simulink model "model_main2"  (R2024b)
settings: Solver=ode4  StartTime=0.0  StopTime=30  FixedStep=0.01  RelTol=1e-3
undefined symbols (not defined in the file): Iws, m_tot, Omega1_init, Omega2_init, Omega3_init, Omega4_init, pI0, qb0, RW_As, SC_Ib, SC_Kepler, TC_Kepler, vI0, wb0
libraries: simulink_extras x3, sharedtransform x2
settings Model: PacingRate=1.100000  Creator=yhj2019  LastModifiedBy=ASCL
settings RTWCC: GPUComputeCapability=3.5

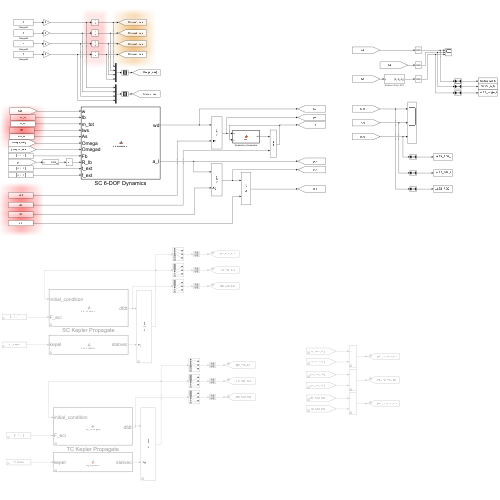
[thumbnail: Simulink's stored preview of the top-level diagram]
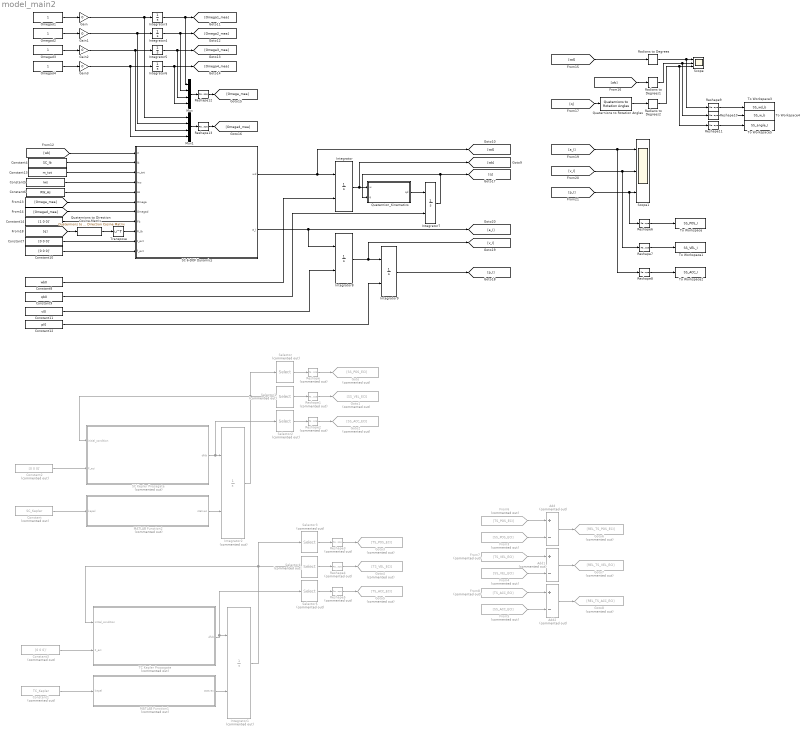
== system model_main2 ==
  Add : Sum  Commented=on  Inputs=+-
  Add1 : Sum  Commented=on  Inputs=+-
  Add2 : Sum  Commented=on  Inputs=+-
  Constant : Constant  Commented=on  Value=SC_Kepler
  Constant1 : Constant  Commented=on  Value=TC_Kepler
  Constant10 : Constant  Value=[0 0 0]'
  Constant11 : Constant  Value=vI0
  Constant12 : Constant  Value=pI0
  Constant13 : Constant  Value=m_tot
  Constant14 : Constant  Value=[1 0 0]'
  Constant2 : Constant  Commented=on  Value=[0 0 0]'
  Constant3 : Constant  Commented=on  Value=[0 0 0]'
  Constant4 : Constant  Value=SC_Ib
  Constant5 : Constant  Value=Iws
  Constant6 : Constant  Value=RW_As
  Constant7 : Constant  Value=[0 0 0]'
  Constant8 : Constant  Value=wb0
  Constant9 : Constant  Value=qb0
  From3 : From  Commented=on  GotoTag=SS_POS_ECI
  From4 : From  Commented=on  GotoTag=SS_VEL_ECI
  From5 : From  Commented=on  GotoTag=SS_ACC_ECI
  From6 : From  Commented=on  GotoTag=TS_POS_ECI
  From7 : From  Commented=on  GotoTag=TS_VEL_ECI
  From8 : From  Commented=on  GotoTag=TS_ACC_ECI
  Gain{,1..3} (4 alike) : Gain  Gain=0
  Goto : Goto  Commented=on  GotoTag=SS_POS_ECI
  Goto1 : Goto  Commented=on  GotoTag=SS_VEL_ECI
  Goto2 : Goto  Commented=on  GotoTag=SS_ACC_ECI
  Goto3 : Goto  Commented=on  GotoTag=TS_POS_ECI
  Goto4 : Goto  Commented=on  GotoTag=TS_VEL_ECI
  Goto5 : Goto  Commented=on  GotoTag=TS_ACC_ECI
  Goto6 : Goto  Commented=on  GotoTag=REL_TS_POS_ECI
  Goto7 : Goto  Commented=on  GotoTag=REL_TS_VEL_ECI
  Goto8 : Goto  Commented=on  GotoTag=REL_TS_ACC_ECI
  Integrator : Integrator  InitialConditionSource=external  InitialCondition=wb0
  Integrator1 : Integrator  Commented=on  InitialConditionSource=external  InitialCondition=[-7000 0 0 0 -9.175045 0 5233.5]'
  Integrator2 : Integrator  Commented=on  InitialConditionSource=external  InitialCondition=[-7000 0 0 0 -9.175045 0 5233.5]'
  Integrator3 : Integrator  InitialCondition=Omega1_init
  Integrator4 : Integrator  InitialCondition=Omega2_init
  Integrator5 : Integrator  InitialCondition=Omega3_init
  Integrator6 : Integrator  InitialCondition=Omega4_init
  Integrator7 : Integrator  InitialConditionSource=external
  Integrator8 : Integrator  InitialConditionSource=external  InitialCondition=wb0
  Integrator9 : Integrator  InitialConditionSource=external  InitialCondition=wb0
  MATLAB Function1 : MATLAB Function  Commented=on  TreatAsAtomicUnit=on
  MATLAB Function2 : MATLAB Function  Commented=on  TreatAsAtomicUnit=on
  Mux : Mux
  Mux1 : Mux
  Omegad{1..4} (4 alike) : Constant
  Quaternion_Kinematics : MATLAB Function  TreatAsAtomicUnit=on
  Quaternions to Direction Cosine Matrix : sharedtransform/Quaternions to  Direction Cosine Matrix  aMode=aMode
      settings: LibrarySourceBlock=|
      | aerolibtransform2/Quaternions to
      | Direction Cosine Matrix
  Quaternions to Rotation Angles : sharedtransform/Quaternions to Rotation Angles  rotationOrder=ZYX  aMode=aMode
  Radians to Degrees : simulink_extras/Transformations/Radians to Degrees
  Radians to Degrees1 : simulink_extras/Transformations/Radians to Degrees
  Radians to Degrees2 : simulink_extras/Transformations/Radians to Degrees
  Reshape{,1..5} (6 alike) : Reshape  Commented=on  OutputDimensionality=Column vector (2-D)
  Reshape{6..11} (6 alike) : Reshape  OutputDimensionality=Row vector (2-D)
  Reshape12 : Reshape  OutputDimensionality=Column vector (2-D)
  Reshape13 : Reshape  OutputDimensionality=Column vector (2-D)
  SC 6-DOF Dynamics : MATLAB Function  TreatAsAtomicUnit=on
  SC Kepler Propagate : MATLAB Function  Commented=on  TreatAsAtomicUnit=on
  Scope : Scope  NumInputPorts=3
  Scope1 : Scope  NumInputPorts=3
  Selector : Selector  Commented=on  InputPortWidth=6  IndexOptions=Index vector (dialog)  Indices=[1 2 3]  OutputSizes=1
  Selector{1..2,4..5} (4 alike) : Selector  Commented=on  InputPortWidth=6  IndexOptions=Index vector (dialog)  Indices=[4 5 6]  OutputSizes=1
  Selector3 : Selector  Commented=on  InputPortWidth=6  IndexOptions=Index vector (dialog)  Indices=[1 2 3]  OutputSizes=1
  TC Kepler Propagate : MATLAB Function  Commented=on  TreatAsAtomicUnit=on
  To Workspace : ToWorkspace  VariableName=SS_POS_I  SampleTime=-1
      settings: Save2DSignal=2-D array (concatenate along first dimension)
  To Workspace1 : ToWorkspace  VariableName=SS_VEL_I  SampleTime=-1
      settings: Save2DSignal=2-D array (concatenate along first dimension)
  To Workspace2 : ToWorkspace  VariableName=SS_ACC_I  SampleTime=-1
      settings: Save2DSignal=2-D array (concatenate along first dimension)
  To Workspace3 : ToWorkspace  VariableName=SS_wd_b  SampleTime=-1
      settings: Save2DSignal=2-D array (concatenate along first dimension)
  To Workspace4 : ToWorkspace  VariableName=SS_w_b  SampleTime=-1
      settings: Save2DSignal=2-D array (concatenate along first dimension)
  To Workspace5 : ToWorkspace  VariableName=SS_angle_I  SampleTime=-1
      settings: Save2DSignal=2-D array (concatenate along first dimension)
  Transpose : Math  Operator=transpose
  wires:
  Constant/1 -> MATLAB Function2/1(kepel)
  Constant1/1 -> MATLAB Function1/1(kepel)
  SC Kepler Propagate/1(dfdt) -> Selector2/1, Integrator2/1
  MATLAB Function2/1(statvec) -> Integrator2/2
  Integrator2/1 -> Selector/1, SC Kepler Propagate/1(initial_condition), Selector1/1
  TC Kepler Propagate/1(dfdt) -> Selector5/1, Integrator1/1
  MATLAB Function1/1(statvec) -> Integrator1/2
  Integrator1/1 -> TC Kepler Propagate/1(initial_condition), Selector4/1, Selector3/1
  Constant2/1 -> SC Kepler Propagate/2(F_eci)
  Constant3/1 -> TC Kepler Propagate/2(F_eci)
  Selector/1 -> Reshape/1
  Selector2/1 -> Reshape2/1
  Selector1/1 -> Reshape1/1
  Reshape/1 -> Goto/1
  Reshape1/1 -> Goto1/1
  Reshape2/1 -> Goto2/1
  Selector5/1 -> Reshape5/1
  Selector4/1 -> Reshape4/1
  Selector3/1 -> Reshape3/1
  Reshape4/1 -> Goto4/1
  Reshape5/1 -> Goto5/1
  Reshape3/1 -> Goto3/1
  Reshape6/1 -> To Workspace/1
  Reshape7/1 -> To Workspace1/1
  Reshape8/1 -> To Workspace2/1
  From6/1 -> Add/1
  From3/1 -> Add/2
  From4/1 -> Add1/2
  From7/1 -> Add1/1
  From5/1 -> Add2/2
  From8/1 -> Add2/1
  Add/1 -> Goto6/1
  Add1/1 -> Goto7/1
  Add2/1 -> Goto8/1
  Constant4/1 -> SC 6-DOF Dynamics/2(Ib)
  Constant5/1 -> SC 6-DOF Dynamics/4(Iws)
  SC 6-DOF Dynamics/1(wd) -> [wd], Integrator/1
  Integrator/1 -> [wb], Quaternion_Kinematics/1(w)
  [wb] -> SC 6-DOF Dynamics/1(w)
  Constant6/1 -> SC 6-DOF Dynamics/5(As)
  Constant7/1 -> SC 6-DOF Dynamics/10(t_ext)
  Omegad1/1 -> Gain/1
  Omegad2/1 -> Gain1/1
  Omegad4/1 -> Gain3/1
  Omegad3/1 -> Gain2/1
  Integrator3/1 -> Mux/1, [Omega1_mea]
  Integrator4/1 -> Mux/2, [Omega2_mea]
  Integrator6/1 -> Mux/4, [Omega4_mea]
  Integrator5/1 -> Mux/3, [Omega3_mea]
  Reshape12/1 -> [Omega_mea]
  Mux/1 -> Reshape12/1
  [Omega_mea] -> SC 6-DOF Dynamics/6(Omega)
  Mux1/1 -> Reshape13/1
  Reshape13/1 -> [Omegad_mea]
  [Omegad_mea] -> SC 6-DOF Dynamics/7(Omegad)
  Quaternion_Kinematics/1(qd) -> Integrator7/1
  Integrator7/1 -> Quaternion_Kinematics/2(q), [q]
  Constant8/1 -> Integrator/2
  Constant9/1 -> Integrator7/2
  Quaternions to Rotation Angles/1 -> Radians to Degrees2/1
  [wd] -> Radians to Degrees/1
  [wb] -> Radians to Degrees1/1
  Radians to Degrees/1 -> Reshape9/1, Scope/1
  Radians to Degrees1/1 -> Reshape10/1, Scope/2
  Radians to Degrees2/1 -> Reshape11/1, Scope/3
  [q] -> Quaternions to Rotation Angles/1
  Constant10/1 -> SC 6-DOF Dynamics/11(f_ext)
  SC 6-DOF Dynamics/2(a_I) -> Integrator8/1, [a_I]
  Constant11/1 -> Integrator8/2
  Constant12/1 -> Integrator9/2
  Integrator8/1 -> [v_I], Integrator9/1
  Constant13/1 -> SC 6-DOF Dynamics/3(m_tot)
  Constant14/1 -> SC 6-DOF Dynamics/8(Fb)
  [q] -> Quaternions to Direction Cosine Matrix/1
  Quaternions to Direction Cosine Matrix/1 -> Transpose/1
  Integrator9/1 -> [p_I]
  [p_I] -> Reshape6/1, Scope1/3
  [v_I] -> Reshape7/1, Scope1/2
  Gain/1 -> Mux1/1, Integrator3/1
  Gain1/1 -> Mux1/2, Integrator4/1
  Gain2/1 -> Mux1/3, Integrator5/1
  Gain3/1 -> Mux1/4, Integrator6/1
  [a_I] -> Reshape8/1, Scope1/1
  Transpose/1 -> SC 6-DOF Dynamics/9(R_Ib)
  Reshape9/1 -> To Workspace3/1
  Reshape10/1 -> To Workspace4/1
  Reshape11/1 -> To Workspace5/1

== matlab function model_main2/MATLAB Function1 ==
  data: kepel input; statvec output
function statvec  = kepel_statvec (kepel)
%  [statvec] = kepel_statvec (kepel)
%	The function kepel_statvec transforms the keplerian
%	elements kepel into the corresponding state vector in
%	the same reference system.
%
% Input:
%	kepel
% 		vector containing the keplerian elements:
%		(1) - semimajor axis of the orbit in meters.
%		(2) - eccentricity.
%		(3) - inclinatsion in radians.
%		(4) - right ascension of ascending node in radians.
%		(5) - argument of perigee in radians.
%		(6) - mean anomaly in radians.
% Output:
%	statvec
%  		state vector in meters and meters/second.
%
% Authors:
%	Helio K. Kuga;
%	Valder M. Medeiros;
%	Valdemir Carrara		february/80		version 1.0
%	Valdemir Carrara		july 2005		(C version)
%   Valdemir Carrara            March/09        Matlab

EARTH_GRAVITY	= 3.9860064e+14;		% Earth's gravitational constant (m**3/s**2)

a    = kepel(1);	% semi-major axis
exc  = kepel(2);	% eccentricity

c1   = sqrt(1. - exc*exc);

%     rotation matrix

orb2iner = rotmaz(-kepel(4))*rotmax(-kepel(3))*rotmaz(-kepel(5));

%     Kepler's equation

E    = kepler(kepel(6), exc);

sE   = sin(E);
cE   = cos(E);
c3   = sqrt(EARTH_GRAVITY/a)/(1. - exc*cE);

%     state vector

statvec = [[a*(cE - exc), a*c1*sE, 0]*orb2iner', [-c3*sE, c1*c3*cE, 0]*orb2iner'];

end

function [rot_mat] = rotmax (angle)
% [rot_mat] = rotmax (angle)
%   To obtain the rotation matrix around the X axis given the
%   rotation angle.
% inputs:
%   angle
%       rotation angle, in radians.
% outputs:
%   rot_mat
%       rotation matrix (3, 3)
%

% Valdemir Carrara, Sep, 1998

coan    =  cos(angle);
sian    =  sin(angle);

rot_mat =  [1, 0, 0; 0, coan, sian; 0, -sian, coan];

end

function [rot_mat] = rotmay (angle)
% [rot_mat] = rotmay (angle)
%   To obtain the rotation matrix around the Y axis given the
%   rotation angle.
% inputs:
%   angle
%       rotation angle, in radians.
% outputs:
%   rot_mat
%       rotation matrix (3, 3)
%

% Valdemir Carrara, Sep, 1998


coan    =  cos(angle);
sian    =  sin(angle);

rot_mat =  [coan, 0, -sian; 0, 1, 0; sian, 0, coan];

end

function [rot_mat] = rotmaz (angle)
% [rot_mat] = rotmaz (angle)
%   To obtain the rotation matrix around the Z axis given the
%   rotation angle.
% inputs:
%   angle
%       rotation angle, in radians.
% outputs:
%   rot_mat
%       rotation matrix (3, 3)
%

% Valdemir Carrara, Sep, 1998

coan    =  cos(angle);
sian    =  sin(angle);

rot_mat =  [coan, sian, 0; -sian, coan, 0; 0, 0, 1];
end

function [eccentric] = kepler (mean_anomaly, eccentricity)
% [eccentric] = kepler (mean_anomaly, eccentricity)
%	The subroutine kepler finds a solution to the
%	kepler's equation.
%
% Input:
%	mean_anomaly
%		mean anomaly in radians.
%	eccentricity
%		eccentricity.
%
% Output:
%	eccentric
%		eccentric anomaly in radians.
%
% Authors:
%	Valder M. de Medeiros		june/81		version 2.0
%	Valdemir Carrara			july 2005	(C version)
%   Valdemir Carrara            March/09        Matlab

exc2    = eccentricity*eccentricity;
am1     = mod (mean_anomaly, 2*pi);
am2     = am1 + am1;
am3     = am1 + am2;
shoot   = am1 + eccentricity*(1. - 0.125*exc2)*sin(am1) + ...
		0.5*exc2*(sin(am2) + 0.75*eccentricity*sin(am3));
shoot   = mod (shoot, 2*pi);

e1      = 1.0;
ic      = 0;

while ((abs(e1) > 1.e-12) && (ic <= 10)) 
	e1    = (shoot - am1 - eccentricity*sin(shoot)) / ...
			(1.0 - eccentricity*cos(shoot));
    shoot = shoot - e1;
    ic    = ic + 1;
end

if (ic >= 10)
    disp ('warning ** subroutine kepler did not converge in 10 iterations');
end

eccentric = shoot;


end

== matlab function model_main2/TC Kepler Propagate ==
  data: initial_condition input; dfdt output; F_eci input
function dfdt  = eq_propagate(initial_condition, F_eci)
% Lectures_TwoBodyProblem.pdf
% 우주시스템입문 - 도미타 노부유키 eq(7.8) p136
% https://en.wikipedia.org/wiki/Standard_gravitational_parameter
u  = 3.9860064e+14; % earth gravitional parameter
Re = 6378137;      % earth radius [m]

dfdt = zeros(size(initial_condition));

% x=x
% x1=dx/dt
% dx1/dt = d^2(x)/dt

x1 = initial_condition(4); % x1 = dx/dt
y1 = initial_condition(5); % y1 = dy/dt
z1 = initial_condition(6); % z1 = dz/dt
x  = initial_condition(1); % x
y  = initial_condition(2); % y
z  = initial_condition(3); % z

r=sqrt(x^2+y^2+z^2);

% % %   Keplar Motion Equatnion
% % %  => r_dd + u/(r^3)r_ = 0 => r_dd = -u/(r^3)r_
dfdt(1) = x1;
dfdt(2) = y1;
dfdt(3) = z1;
dfdt(4) = -u*x/(r^3) + F_eci(1);
dfdt(5) = -u*y/(r^3) + F_eci(2);
dfdt(6) = -u*z/(r^3) + F_eci(3);

end

== matlab function model_main2/SC 6-DOF Dynamics ==
  data: w input; Ib input; m_tot input; wd output; Iws input; As input; Omega input; Omegad input; Fb input; R_Ib input; t_ext input; f_ext input; a_I output
function [wd, a_I]  = eq_propagate(w, Ib, m_tot, ...
                                                  Iws, As, Omega, Omegad, ...
                                                  Fb, R_Ib, ...
                                                  t_ext, f_ext)
% % 
% 출력 1: 위성 동체 좌표계 각가속도
% 출력 2: 관성좌표계 선가속도


RW_h = As*Iws*Omega;
RW_hd = As*Iws*Omegad;

%% Rotational Motion
wd = inv(Ib)*(t_ext - RW_hd - cross(w, Ib*w + RW_h));

%% Translational Motion

a_I = (R_Ib*Fb + f_ext)/m_tot;

end

== matlab function model_main2/SC Kepler Propagate ==
  data: initial_condition input; dfdt output; F_eci input
function dfdt  = eq_propagate(initial_condition, F_eci)
% Lectures_TwoBodyProblem.pdf
% 우주시스템입문 - 도미타 노부유키 eq(7.8) p136
% https://en.wikipedia.org/wiki/Standard_gravitational_parameter
u  = 3.9860064e+14; % earth gravitional parameter
Re = 6378137;      % earth radius [m]

dfdt = zeros(size(initial_condition));

% x=x
% x1=dx/dt
% dx1/dt = d^2(x)/dt

x1 = initial_condition(4); % x1 = dx/dt
y1 = initial_condition(5); % y1 = dy/dt
z1 = initial_condition(6); % z1 = dz/dt
x  = initial_condition(1); % x
y  = initial_condition(2); % y
z  = initial_condition(3); % z

r=sqrt(x^2+y^2+z^2);

% % %   Keplar Motion Equatnion
% % %  => r_dd + u/(r^3)r_ = 0 => r_dd = -u/(r^3)r_
dfdt(1) = x1;
dfdt(2) = y1;
dfdt(3) = z1;
dfdt(4) = -u*x/(r^3) + F_eci(1);
dfdt(5) = -u*y/(r^3) + F_eci(2);
dfdt(6) = -u*z/(r^3) + F_eci(3);

end

== matlab function model_main2/MATLAB Function2 ==
  data: kepel input; statvec output
function statvec  = kepel_statvec (kepel)
%  [statvec] = kepel_statvec (kepel)
%	The function kepel_statvec transforms the keplerian
%	elements kepel into the corresponding state vector in
%	the same reference system.
%
% Input:
%	kepel
% 		vector containing the keplerian elements:
%		(1) - semimajor axis of the orbit in meters.
%		(2) - eccentricity.
%		(3) - inclinatsion in radians.
%		(4) - right ascension of ascending node in radians.
%		(5) - argument of perigee in radians.
%		(6) - mean anomaly in radians.
% Output:
%	statvec
%  		state vector in meters and meters/second.
%
% Authors:
%	Helio K. Kuga;
%	Valder M. Medeiros;
%	Valdemir Carrara		february/80		version 1.0
%	Valdemir Carrara		july 2005		(C version)
%   Valdemir Carrara            March/09        Matlab

EARTH_GRAVITY	= 3.9860064e+14;		% Earth's gravitational constant (m**3/s**2)

a    = kepel(1);	% semi-major axis
exc  = kepel(2);	% eccentricity

c1   = sqrt(1. - exc*exc);

%     rotation matrix

orb2iner = rotmaz(-kepel(4))*rotmax(-kepel(3))*rotmaz(-kepel(5));

%     Kepler's equation

E    = kepler(kepel(6), exc);

sE   = sin(E);
cE   = cos(E);
c3   = sqrt(EARTH_GRAVITY/a)/(1. - exc*cE);

%     state vector

statvec = [[a*(cE - exc), a*c1*sE, 0]*orb2iner', [-c3*sE, c1*c3*cE, 0]*orb2iner'];

end

function [rot_mat] = rotmax (angle)
% [rot_mat] = rotmax (angle)
%   To obtain the rotation matrix around the X axis given the
%   rotation angle.
% inputs:
%   angle
%       rotation angle, in radians.
% outputs:
%   rot_mat
%       rotation matrix (3, 3)
%

% Valdemir Carrara, Sep, 1998

coan    =  cos(angle);
sian    =  sin(angle);

rot_mat =  [1, 0, 0; 0, coan, sian; 0, -sian, coan];

end

function [rot_mat] = rotmay (angle)
% [rot_mat] = rotmay (angle)
%   To obtain the rotation matrix around the Y axis given the
%   rotation angle.
% inputs:
%   angle
%       rotation angle, in radians.
% outputs:
%   rot_mat
%       rotation matrix (3, 3)
%

% Valdemir Carrara, Sep, 1998


coan    =  cos(angle);
sian    =  sin(angle);

rot_mat =  [coan, 0, -sian; 0, 1, 0; sian, 0, coan];

end

function [rot_mat] = rotmaz (angle)
% [rot_mat] = rotmaz (angle)
%   To obtain the rotation matrix around the Z axis given the
%   rotation angle.
% inputs:
%   angle
%       rotation angle, in radians.
% outputs:
%   rot_mat
%       rotation matrix (3, 3)
%

% Valdemir Carrara, Sep, 1998

coan    =  cos(angle);
sian    =  sin(angle);

rot_mat =  [coan, sian, 0; -sian, coan, 0; 0, 0, 1];
end

function [eccentric] = kepler (mean_anomaly, eccentricity)
% [eccentric] = kepler (mean_anomaly, eccentricity)
%	The subroutine kepler finds a solution to the
%	kepler's equation.
%
% Input:
%	mean_anomaly
%		mean anomaly in radians.
%	eccentricity
%		eccentricity.
%
% Output:
%	eccentric
%		eccentric anomaly in radians.
%
% Authors:
%	Valder M. de Medeiros		june/81		version 2.0
%	Valdemir Carrara			july 2005	(C version)
%   Valdemir Carrara            March/09        Matlab

exc2    = eccentricity*eccentricity;
am1     = mod (mean_anomaly, 2*pi);
am2     = am1 + am1;
am3     = am1 + am2;
shoot   = am1 + eccentricity*(1. - 0.125*exc2)*sin(am1) + ...
		0.5*exc2*(sin(am2) + 0.75*eccentricity*sin(am3));
shoot   = mod (shoot, 2*pi);

e1      = 1.0;
ic      = 0;

while ((abs(e1) > 1.e-12) && (ic <= 10)) 
	e1    = (shoot - am1 - eccentricity*sin(shoot)) / ...
			(1.0 - eccentricity*cos(shoot));
    shoot = shoot - e1;
    ic    = ic + 1;
end

if (ic >= 10)
    disp ('warning ** subroutine kepler did not converge in 10 iterations');
end

eccentric = shoot;


end

== matlab function model_main2/Quaternion_Kinematics ==
  data: w input; qd output; q input
function qd = fcn(w,q)

F_q = (1/2)*[0 -w(1) -w(2) -w(3);
       w(1) 0 w(3) -w(2);
       w(2) -w(3) 0 w(1);
       w(3) w(2) -w(1) 0];

qd = F_q*q;

end
